simulink model "Project2b"  (R2015b)
settings: Solver=ode45  StartTime=0.0  StopTime=5  FixedStep=0.001  RelTol=1e-3
values from neighbouring files (symbols this model uses):
  x1e = z(1)    [Project2full.m]
  x2e = z(2)    [Project2full.m]
settings Model: Creator=Dell  LastModifiedBy=Dell
settings DataIOCC: LimitDataPoints=off

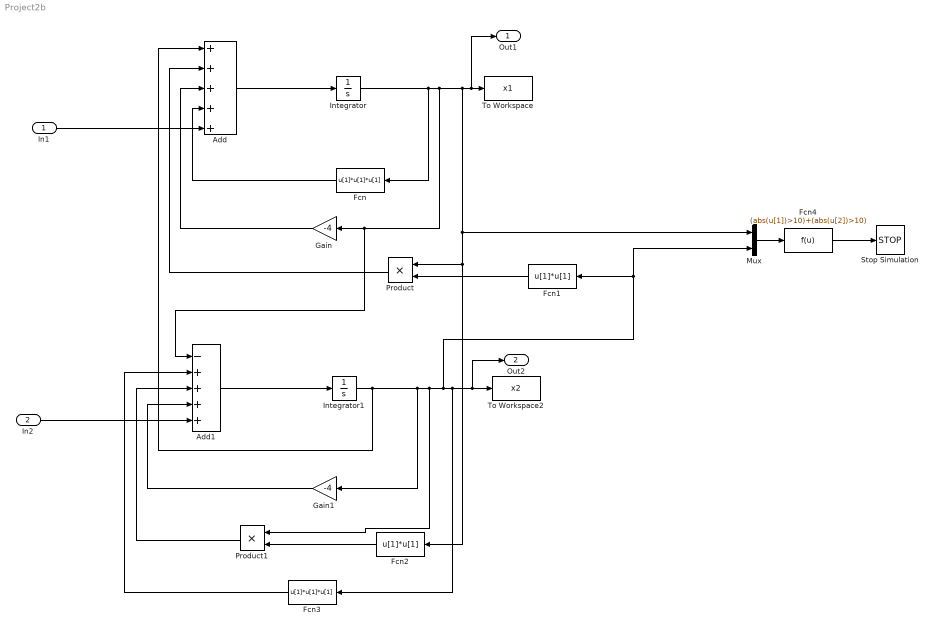
== system Project2b ==
  In1 : Inport
  In2 : Inport  Port=2
  Add : Sum  Inputs=+++++
  Add1 : Sum  Inputs=-++++
  Fcn : Fcn  Expr=u[1]*u[1]*u[1]
  Fcn1 : Fcn  Expr=u[1]*u[1]
  Fcn2 : Fcn  Expr=u[1]*u[1]
  Fcn3 : Fcn  Expr=u[1]*u[1]*u[1]
  Fcn4 : Fcn  Expr=(abs(u[1])>10)+(abs(u[2])>10)
  Gain : Gain  Gain=-4
  Gain1 : Gain  Gain=-4
  Integrator : Integrator  InitialCondition=x1e
  Integrator1 : Integrator  InitialCondition=x2e
  Mux : Mux  Inputs=2
  Product : Product
  Product1 : Product
  Stop Simulation : Stop
  To Workspace : ToWorkspace  VariableName=x1  SampleTime=-1
  To Workspace2 : ToWorkspace  VariableName=x2  SampleTime=-1
  Out1 : Outport
  Out2 : Outport  Port=2
  wires:
  Add/1 -> Integrator/1
  Integrator/1 -> Fcn/1, Add1/1, Gain/1, Mux/1, Fcn2/1, Product/1, Out1/1, To Workspace/1
  Add1/1 -> Integrator1/1
  Integrator1/1 -> Add/1, Gain1/1, Product1/1, Mux/2, Fcn1/1, Fcn3/1, Out2/1, To Workspace2/1
  Fcn/1 -> Add/4
  Gain/1 -> Add/3
  Fcn1/1 -> Product/2
  Product/1 -> Add/2
  Fcn2/1 -> Product1/2
  Product1/1 -> Add1/3
  Gain1/1 -> Add1/4
  Fcn3/1 -> Add1/2
  Mux/1 -> Fcn4/1
  Fcn4/1 -> Stop Simulation/1
  In1/1 -> Add/5
  In2/1 -> Add1/5
